simulink model "Problem2"  (R2020a)
settings: Solver=VariableStepAuto  StartTime=0.0  StopTime=100  MaxStep=0.01  RelTol=1e-3
settings Model: Creator=Shreyas  LastModifiedBy=Shreyas

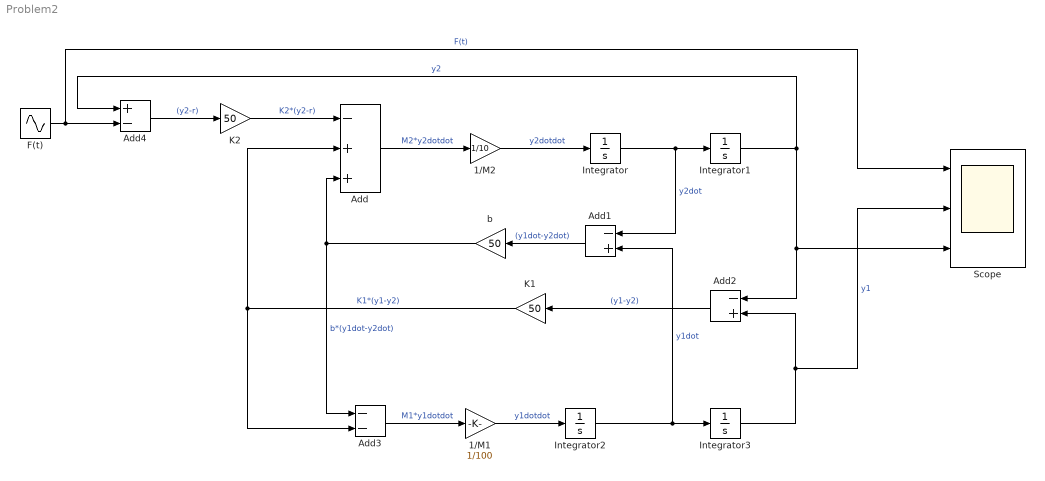
== system Problem2 ==
  1/M1 : Gain  Gain=1/100
  1/M2 : Gain  Gain=1/10
  Add : Sum  Inputs=-++
  Add1 : Sum  Inputs=-+
  Add2 : Sum  Inputs=-+
  Add3 : Sum  Inputs=--
  Add4 : Sum  Inputs=+-
  F(t) : Sin  SampleTime=0
  Integrator{,1..3} (4 alike) : Integrator
  K1 : Gain  Gain=50
  K2 : Gain  Gain=50
  Scope : Scope  NumInputPorts=3
  b : Gain  Gain=50
  wires:
  Add/1 -> 1/M2/1  "M2*y2dotdot"
  1/M2/1 -> Integrator/1  "y2dotdot"
  Integrator/1 -> Add1/1, Integrator1/1  "y2dot"
  Add1/1 -> b/1  "(y1dot-y2dot)"
  Add2/1 -> K1/1  "(y1-y2)"
  1/M1/1 -> Integrator2/1  "y1dotdot"
  Add3/1 -> 1/M1/1  "M1*y1dotdot"
  Integrator2/1 -> Add1/2, Integrator3/1  "y1dot"
  Integrator3/1 -> Add2/2, Scope/2  "y1"
  Integrator1/1 -> Add2/1, Scope/3, Add4/1  "y2"
  b/1 -> Add3/1, Add/3  "b*(y1dot-y2dot)"
  K1/1 -> Add3/2, Add/2  "K1*(y1-y2)"
  F(t)/1 -> Scope/1, Add4/2  "F(t)"
  Add4/1 -> K2/1  "(y2-r)"
  K2/1 -> Add/1  "K2*(y2-r)"
